simulink model "Operators"  (R2024a)
settings: Solver=FixedStepDiscrete  StartTime=0.0  StopTime=10.0  FixedStep=1e-3  RelTol=1e-3
settings Model: Creator=VICTUS  LastModifiedBy=VICTUS

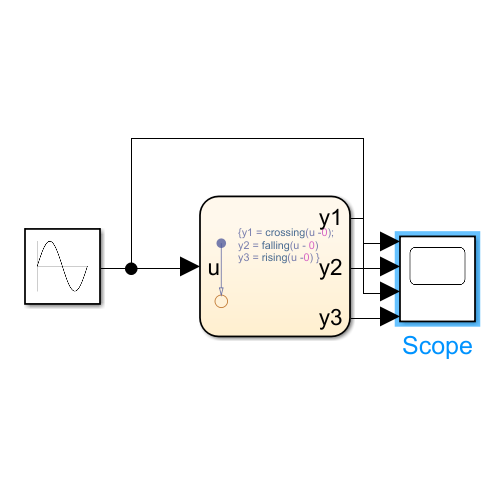
[thumbnail: Simulink's stored preview of the top-level diagram]
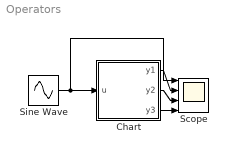
== system Operators ==
  Chart : Stateflow chart  TreatAsAtomicUnit=on
  Scope : Scope  NumInputPorts=4
  Sine Wave : Sin  SampleTime=0
  wires:
  Sine Wave/1 -> Scope/1, Chart/1(u)
  Chart/1(y1) -> Scope/2
  Chart/2(y2) -> Scope/3
  Chart/3(y3) -> Scope/4

== stateflow chart Operators/Chart ==
  (default) -> (junction 1) : {y1 = crossing(u -0);
      | y2 = falling(u - 0)
      | y3 = rising(u -0) }
  data: u input; y1 output; y2 output; y3 output
